simulink model "FYP"  (R2023b)
settings: Solver=FixedStepAuto  StartTime=0.0  StopTime=Inf  RelTol=1e-3  EnableMultiTasking=on
libraries: canmsglib x26, raspberrypiCommlib x26
(part 4 of 4)

== matlab function FYP/BMS Energy Status/MATLAB Function1 ==
  data: soc input; remainingEnergy output
function remainingEnergy = fcn(soc)

socdec = soc/100;
invdec = 1/socdec;

remainingEnergy = 75*invdec;

== matlab function FYP/Average Voltage ==
  data: v1 input; v output; v2 input; v3 input; v4 input
function v = fcn(v1,v2,v3,v4)

v = mean([v1*(23/96),v2*(25/96),v3*(25/96),v4*(23/96)]);

== matlab function FYP/Average Temp ==
  data: v1 input; v output; v2 input; v3 input; v4 input
function v = fcn(v1,v2,v3,v4)

v = mean([v1,v2,v3,v4]);

== matlab function FYP/Power Distr ==
  data: pr input; p1 output; p2 output; p3 output; p4 output
function [p1,p2,p3,p4] = fcn(pr)

p1 = (23/96)*pr;
p4 = p1;

p2 = (25/96)*pr;
p3 = p2;

== matlab function FYP/Coolant Dist ==
  data: pr input; p1 output; p2 output; p3 output; p4 output
function [p1,p2,p3,p4] = fcn(pr)

p1 = (23/96)*pr;
p4 = p1;

p2 = (25/96)*pr;
p3 = p2;

== matlab function FYP/Sys Time ==
  data: trigger input; day output; hour output; minute output; month output; second output; year output
function [day, hour, minute, month, second, year] = fcn(trigger)

utcTime = datetime('now');

day = utcTime.Day;
hour = utcTime.Hour;
minute = utcTime.Minute;
month = utcTime.Month;
second = utcTime.Second;
year = utcTime.Year;

== matlab function FYP/BMS Module State Monitoring/MATLAB Function ==
  data: m1 input; maxV output; maxIdx output; m2 input; m3 input; m4 input; minV output; minIdx output
function [maxV, maxIdx, minV, minIdx] = findMaxMin(m1, m2, m3, m4)
    values = [m1, m2, m3, m4];
    
    [maxV, maxIdx] = max(values);
    [minV, minIdx] = min(values);
end

== matlab function FYP/BMS Module State Monitoring/MATLAB Function1 ==
  data: m1 input; maxT output; maxIdx output; m2 input; m3 input; m4 input; minT output; minIdx output
function [maxT, maxIdx, minT, minIdx] = findMaxMin(m1, m2, m3, m4)
    values = [m1, m2, m3, m4];
    
    [maxT, maxIdx] = max(values);
    [minT, minIdx] = min(values);
end

== matlab function FYP/MATLAB Function2 ==
  data: currentW input; percent output
function percent = energyPercentage(currentW)

    if currentW == 0
        percent = 0;
    else
        maxW = 393000;
        percent = (currentW / maxW) * 100;
    end
end

== matlab function FYP/MATLAB Function3 ==
  data: Range output; Energy input
function Range   = fcn( Energy)

Range = Energy*4.8;

== matlab function FYP/MATLAB Function4 ==
  data: vehicle_speed_mps input; power_W output; motor_torque_Nm input; rolling_radius_m input
function power_W = computeMotorPower(vehicle_speed_mps, motor_torque_Nm, rolling_radius_m)
% computeMotorPower - Calculates motor power based on vehicle speed, torque, radius, and gear ratio.
%
% Inputs:
%   vehicle_speed_mps   - Vehicle speed in meters per second (m/s)
%   motor_torque_Nm     - Motor torque in newton-meters (Nm)
%   rolling_radius_m    - Rolling radius of the wheel in meters (m)
%   gear_ratio          - Gear ratio (motor speed / wheel speed)
%
% Output:
%   power_W             - Motor power in watts (W)

    % Step 1: Angular velocity of wheel
    omega_wheel = vehicle_speed_mps / rolling_radius_m;  % rad/s

    % Step 2: Angular velocity of motor
    omega_motor = omega_wheel * 9.03;  % rad/s

    % Step 3: Power
    power_W = motor_torque_Nm * omega_motor;  % Watts
end

== matlab function FYP/MATLAB Function5 ==
  data: vehicle_speed_mps input; power_W output; motor_torque_Nm input; rolling_radius_m input
function power_W = computeMotorPower(vehicle_speed_mps, motor_torque_Nm, rolling_radius_m)
% computeMotorPower - Calculates motor power based on vehicle speed, torque, radius, and gear ratio.
%
% Inputs:
%   vehicle_speed_mps   - Vehicle speed in meters per second (m/s)
%   motor_torque_Nm     - Motor torque in newton-meters (Nm)
%   rolling_radius_m    - Rolling radius of the wheel in meters (m)
%
% Output:
%   power_W             - Motor power in watts (W)

    % Step 1: Angular velocity of wheel
    omega_wheel = vehicle_speed_mps / rolling_radius_m;  % rad/s

    % Step 2: Angular velocity of motor
    omega_motor = omega_wheel * 9.03;  % rad/s

    % Step 3: Power
    power_W = motor_torque_Nm * omega_motor;  % Watts
end

== matlab function FYP/MATLAB Function ==
  data: charge output; power input; discharge output
function [charge, discharge] = fcn(power)

    % Default assignments to prevent unassigned error
    charge = 0;
    discharge = 0;

    if power <= 0
        discharge = abs(power);
    elseif power > 0
        charge = power;
    end
end

== matlab function FYP/Rear PT Kinematics/checksum calc ==
  data: data input; chcksm output
function chcksm = fcn(data)

data = uint8(data);
total = sum(data);
chcksm =  mod(total,256);

== matlab function FYP/Rear PT Kinematics/MATLAB Function ==
  data: counter input; newCounter output
function newCounter = incrementCounter(counter)
    newCounter = mod(counter + 1, 16);

== matlab function FYP/Rear PT Torque/MATLAB Function ==
  data: counter input; newCounter output
function newCounter = incrementCounter(counter)
    newCounter = mod(counter + 1, 8);

== matlab function FYP/Rear PT Torque/checksum calc ==
  data: data input; chcksm output
function chcksm = fcn(data)

data = uint8(data);
total = sum(data);
chcksm =  mod(total,256);

== matlab function FYP/Front PT Kinematics/MATLAB Function ==
  data: counter input; newCounter output
function newCounter = incrementCounter(counter)
    newCounter = mod(counter + 1, 16);

== matlab function FYP/Front PT Kinematics/checksum calc ==
  data: data input; chcksm output
function chcksm = fcn(data)

data = uint8(data);
total = sum(data);
chcksm =  mod(total,256);

== matlab function FYP/Front PT Kinematics/m//s to RPM ==
  data: vSpeed input; rpm output; R input
function rpm = fcn(vSpeed,R)

rpm = (vSpeed*60)/(2*pi*R);

== matlab function FYP/Unix Time ==
  data: trigger input; UnixTime output
function UnixTime = fcn(trigger)

utcTime = datetime('now');
UnixTime = posixtime(utcTime);

== matlab function FYP/MATLAB Function1 ==
  data: accelPct input; torqueFront output; brakePct input; torqueRear output; PRND input; soc input; motorSpeedRadPerSec input
function [torqueFront, torqueRear] = MATLAB_Function1(accelPct, brakePct, PRND, soc, motorSpeedRadPerSec)
% motorController - Calculates front and rear motor torques based on pedal inputs and gear selection
%
% Inputs:
%   accelPct           - Accelerator pedal percentage (0-100)
%   brakePct           - Brake pedal percentage (0-100)
%   PRND               - Gear selector: 0 = Park, 1 = Reverse, 2 = Neutral, 3 = Drive
%   soc                - State of charge
%   motorSpeedRadPerSec - Current motor speed (rad/s)
%
% Outputs:
%   torqueFront - Requested torque for the front motor (Nm)
%   torqueRear  - Requested torque for the rear motor (Nm)

    frontSplit = 0.363;

    % Constants
    maxDriveTorque = 660;      % Nm
    maxRegenTorque = -660;     % Nm
    maxPowerFront = 393000*frontSplit;     % W (hardcoded max front motor power)
    maxPowerRear  = 393000-maxPowerFront;     % W (hardcoded max rear motor power)

    % Clamp inputs
    accelPct = max(0, min(accelPct, 100));
    brakePct = max(0, min(brakePct, 100));

    % Initialize torque
    totalTorque = 0;

    % Compute total torque based on gear and pedal inputs
    if PRND == 3  % Drive
        if brakePct > 0
            totalTorque = (brakePct / 100) * maxRegenTorque;
        elseif accelPct > 0
            totalTorque = (accelPct / 100) * maxDriveTorque;
        end
    elseif PRND == 1  % Reverse
        if brakePct > 0
            totalTorque = -1 * (brakePct / 100) * maxRegenTorque;
        elseif accelPct > 0
            totalTorque = -1 * (accelPct / 100) * maxDriveTorque;
        end
    end

    % Apply front/rear split
    torqueFront = frontSplit * totalTorque;
    torqueRear  = (1 - frontSplit) * totalTorque;

    % Limit power for front motor
    powerFront = abs(torqueFront * motorSpeedRadPerSec);
    if powerFront > maxPowerFront
        torqueFront = torqueFront * (maxPowerFront / powerFront);
    end

    % Limit power for rear motor
    powerRear = abs(torqueRear * motorSpeedRadPerSec);
    if powerRear > maxPowerRear
        torqueRear = torqueRear * (maxPowerRear / powerRear);
    end

    % SOC check
    if soc <= 0
        torqueFront = 0;
        torqueRear = 0;
    end
end

== matlab function FYP/Coastdown Func ==
  data: v input; F_total output
function F_total = coastdown_force(v)
% COASTDOWN_FORCE Calculates coastdown force for a Tesla Model 3 Performance
%
%   F_total = COASTDOWN_FORCE(v)
%
%   Input:
%       v - Vehicle speed in m/s (scalar or vector)
%
%   Output:
%       F_total - Total coastdown force [N]

    % Parameters for Tesla Model 3 Performance
    rho = 1.2;       % Air density [kg/m^3]
    Cd  = 0.219;        % Drag coefficient
    A   = 2.22;        % Frontal area [m^2]
    m   = 2171;        % Vehicle mass [kg]
    g   = 9.81;        % Gravity [m/s^2]

    % Speed-dependent rolling resistance coefficients
    a = 0.0025;        % [1/m]
    b = 0.0063;         % unitless

    % Aerodynamic drag
    F_aero = 0.5 * rho * Cd * A * v.^2;

    % Speed-dependent rolling resistance
    F_roll = (a * v + b) * m * g;

    % Total coastdown force
    F_total = F_aero + F_roll;

    % Set force to zero where speed is less than 0.01
    F_total(v < 0.1) = 0;
end

== matlab function FYP/Vehicle Estimates/MATLAB Function ==
  data: counter input; newCounter output
function newCounter = incrementCounter(counter)
    newCounter = mod(counter + 1, 8);

== matlab function FYP/Vehicle Estimates/checksum calc ==
  data: data input; chcksm output
function chcksm = fcn(data)

data = uint8(data);
total = sum(data);
chcksm =  mod(total,256);

== matlab function FYP/Subsystem1/MATLAB Function ==
  data: counter input; newCounter output
function newCounter = incrementCounter(counter)
    newCounter = mod(counter + 1, 8);

== matlab function FYP/Subsystem1/checksum calc ==
  data: data input; chcksm output
function chcksm = fcn(data)

data = uint8(data);
total = sum(data);
chcksm =  mod(total,256);

== matlab function FYP/Subsystem1/MATLAB Function1 ==
  data: Speed output; v input; hsSpeed output
function [Speed,hsSpeed] = UISpeeds(v)

Speed = v*1.02;
hsSpeed = v*1.03;

== matlab function FYP/Range Estimations/MATLAB Function ==
  data: SOC input; Range output; SOC output; idealRange output; WHpM output; uSOE output; Energy input
function [Range, SOC, idealRange, WHpM, uSOE]  = fcn(SOC, Energy)

uSOE = SOC;

Range = Energy*4.84;
idealRange = Energy*5.98;

WHpM = 332;

== matlab function FYP/Elevation ==
  data: trigger input; Elevation output
function Elevation = fcn(trigger)

% Elevation assumed to be constant, chosen value from elevation of MIRA.
Elevation = 99;

== matlab function FYP/VIN Generation ==
  data: trigger input; VINA output; VINB output; VINC output; MUX output; VINA2 output; VINB2 output; VINC2 output
function [VINA,VINB,VINC,MUX,VINA2,VINB2,VINC2] = fcn(trigger)

% VIN = 'LRW3F7EL9PC774549';
% 
% VINB = double(VIN(11:17));
% VINC = double(VIN(4:10));
% VINA = double([0, 0, 0, 0, VIN(1:3)]);

VINA = 48484848;
VINB = 67555552;
VINC = 51705569;
MUX = 16;

VINA2 = 768287;
VINB2 = 535257;
VINC2 = 765780;

== matlab function FYP/VIN Generation1 ==
  data: trigger input; VINA output; VINB output; VINC output; MUX output; VINA2 output; VINB2 output; VINC2 output
function [VINA,VINB,VINC,MUX,VINA2,VINB2,VINC2] = fcn(trigger)

% VIN = 'LRW3F7EL9PC774549';
% 
% VINB = double(VIN(11:17));
% VINC = double(VIN(4:10));
% VINA = double([0, 0, 0, 0, VIN(1:3)]);

VINA = 48484848;
VINB = 67555552;
VINC = 51705569;
MUX = 17;

VINA2 = 768287;
VINB2 = 535257;
VINC2 = 765780;

== matlab function FYP/VIN Generation2 ==
  data: trigger input; VINA output; VINB output; VINC output; MUX output; VINA2 output; VINB2 output; VINC2 output
function [VINA,VINB,VINC,MUX,VINA2,VINB2,VINC2] = fcn(trigger)

% VIN = 'LRW3F7EL9PC774549';
% 
% VINB = double(VIN(11:17));
% VINC = double(VIN(4:10));
% VINA = double([0, 0, 0, 0, VIN(1:3)]);

VINA = 48484848;
VINB = 67555552;
VINC = 51705569;
MUX = 18;

VINA2 = 768287;
VINB2 = 535257;
VINC2 = 765780;

== matlab function FYP/BMS SOC/deg to % ==
  data: battTempC input; battTempPct output
function battTempPct = batteryTempDegtoPct(battTempC)

T_min = -20;
T_max = 60;

battTempPct = ((battTempC - T_min) / (T_max - T_min)) * 100;

== matlab function FYP/Rear PT Kinematics/m//s to RPM ==
  data: vSpeed input; rpm output; R input
function rpm = fcn(vSpeed,R)

rpm = (vSpeed*60)/(2*pi*R);

== matlab function FYP/BMS Energy Status/MATLAB Function ==
  data: soc input; bool output
function bool = fcn(soc)

if soc >= 100
    bool = 1;
else
    bool = 0;
end
